simulink model "BiCopter_Landing"  (R2024a)
settings: Solver=ode4  StartTime=0.0  StopTime=20  FixedStep=0.005  RelTol=1e-3
values from neighbouring files (symbols this model uses):
  k = lqr(A,B,Q,R)    [K_Mat.m]    (also in R_good.mat = [-3.51546428725e-11 5.71513441117e-12 1000 1.44018719859e-11)
libraries: simulink_extras x6, shared6dof x3, fuzblock x3
settings Model: Creator=moham  LastModifiedBy=sepehrmahfar
settings OptimizationCC: ReuseModelBlockBuffer=off
settings RTWCC: GPUComputeCapability=3.5

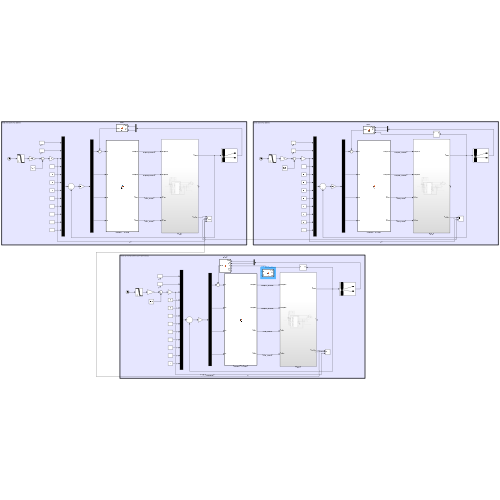
[thumbnail: Simulink's stored preview of the top-level diagram]
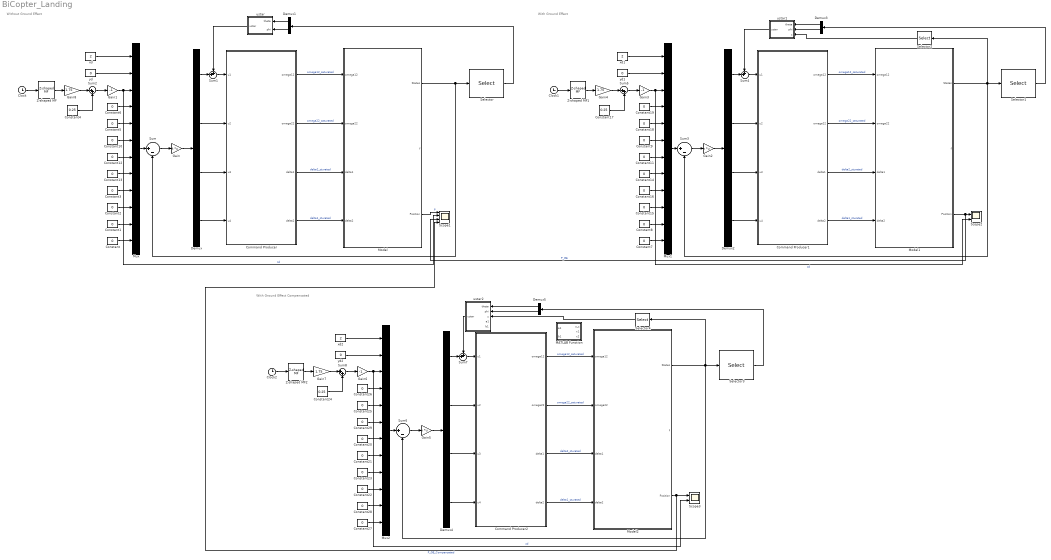
== system BiCopter_Landing ==
  note: Without Ground Effect
  note: With Ground Effect
  note: With Ground Effect Compensated
  Clock : Clock
  Clock1 : Clock
  Clock2 : Clock
  Command Producer : MATLAB Function  TreatAsAtomicUnit=on
  Command Producer1 : MATLAB Function  TreatAsAtomicUnit=on
  Command Producer2 : MATLAB Function  TreatAsAtomicUnit=on
  Constant{,1..3,5..16,18..23,25..29} (27 alike) : Constant  Value=0
  Constant17 : Constant  Value=0.25
  Constant24 : Constant  Value=0.25
  Constant4 : Constant  Value=0.25
  Demux : Demux
  Demux1 : Demux  Outputs=2
  Demux2 : Demux
  Demux3 : Demux  Outputs=2
  Demux4 : Demux
  Demux5 : Demux  Outputs=2
  Gain : Gain  Gain=k  Multiplication=Matrix(K*u)
  Gain1 : Gain  Gain=-1
  Gain2 : Gain  Gain=k  Multiplication=Matrix(K*u)
  Gain3 : Gain  Gain=-1
  Gain4 : Gain  Gain=1.75
  Gain5 : Gain  Gain=k  Multiplication=Matrix(K*u)
  Gain6 : Gain  Gain=-1
  Gain7 : Gain  Gain=1.75
  Gain8 : Gain  Gain=1.75
  MATLAB Function : MATLAB Function  TreatAsAtomicUnit=on
  Model : Subsystem
  Model1 : Subsystem
  Model2 : Subsystem
  Mux : Mux  Inputs=12
  Mux1 : Mux  Inputs=12
  Mux2 : Mux  Inputs=12
  Scope1 : Scope  NumInputPorts=4
  Scope2 : Scope  NumInputPorts=2
  Scope3 : Scope  NumInputPorts=2
  Selector : Selector  InputPortWidth=12  IndexOptions=Index vector (dialog)  Indices=[7 8]  OutputSizes=1
  Selector1 : Selector  InputPortWidth=12  IndexOptions=Index vector (dialog)  Indices=[7 8]  OutputSizes=1
  Selector2 : Selector  InputPortWidth=12  IndexOptions=Index vector (dialog)  Indices=3  OutputSizes=1
  Selector3 : Selector  InputPortWidth=12  IndexOptions=Index vector (dialog)  Indices=[7 8]  OutputSizes=1
  Selector4 : Selector  InputPortWidth=12  IndexOptions=Index vector (dialog)  Indices=3  OutputSizes=1
  Sum : Sum  Inputs=|+-
  Sum1 : Sum  Inputs=++|
  Sum2 : Sum  Inputs=|++
  Sum3 : Sum  Inputs=|+-
  Sum4 : Sum  Inputs=++|
  Sum5 : Sum  Inputs=|++
  Sum6 : Sum  Inputs=|+-
  Sum7 : Sum  Inputs=++|
  Sum8 : Sum  Inputs=|++
  Z-shaped MF : fuzblock/Membership  Functions/Z-shaped MF  a=10  b=15
  Z-shaped MF1 : fuzblock/Membership  Functions/Z-shaped MF  a=10  b=15
  Z-shaped MF2 : fuzblock/Membership  Functions/Z-shaped MF  a=10  b=15
  ustar : MATLAB Function  TreatAsAtomicUnit=on
  ustar1 : MATLAB Function  TreatAsAtomicUnit=on
  ustar2 : MATLAB Function  TreatAsAtomicUnit=on
  xd : Constant  Value=2
  xd1 : Constant  Value=2
  xd2 : Constant  Value=2
  yd : Constant  Value=0
  yd1 : Constant  Value=0
  yd2 : Constant  Value=0
  wires:
  Constant/1 -> Mux/12
  Model/1(States) -> Selector/1, Sum/2
  Mux/1 -> Sum/1
  Constant1/1 -> Mux/11
  Constant2/1 -> Mux/10
  Constant6/1 -> Mux/4
  Constant5/1 -> Mux/5
  Constant10/1 -> Mux/6
  Gain1/1 -> Scope1/2, Mux/3  "zd"
  Command Producer/4(delta2) -> Model/4(delta2)  "delta1_sturated"
  Command Producer/3(delta1) -> Model/3(delta1)  "delta2_sturated"
  Command Producer/2(omega22) -> Model/2(omega22)  "omega22_saturated"
  Command Producer/1(omega12) -> Model/1(omega12)  "omega12_saturated"
  Demux/4 -> Command Producer/4(u4)
  Demux/3 -> Command Producer/3(u3)
  Demux/2 -> Command Producer/2(u2)
  ustar/1(ustar) -> Sum1/1
  Constant12/1 -> Mux/7
  Constant13/1 -> Mux/8
  Sum/1 -> Gain/1
  Gain/1 -> Demux/1
  xd/1 -> Mux/1
  yd/1 -> Mux/2
  Selector/1 -> Demux1/1
  Demux1/2 -> ustar/2(phi)
  Demux1/1 -> ustar/1(theta)
  Model/3(Position) -> Scope1/1  "P"
  Constant3/1 -> Mux/9
  Sum1/1 -> Command Producer/1(u1)
  Demux/1 -> Sum1/2
  Gain8/1 -> Sum2/1
  Clock/1 -> Z-shaped MF/1
  Constant4/1 -> Sum2/2
  Z-shaped MF/1 -> Gain8/1
  Sum2/1 -> Gain1/1
  Demux3/1 -> ustar1/1(theta)
  Constant16/1 -> Mux1/9
  Gain2/1 -> Demux2/1
  Selector1/1 -> Demux3/1
  Model1/3(Position) -> Scope1/3, Scope2/1  "P_GE"
  xd1/1 -> Mux1/1
  Demux3/2 -> ustar1/2(phi)
  Constant19/1 -> Mux1/4
  Constant11/1 -> Mux1/7
  Command Producer1/4(delta2) -> Model1/4(delta2)  "delta1_sturated"
  ustar1/1(ustar) -> Sum4/1
  Constant18/1 -> Mux1/5
  Demux2/3 -> Command Producer1/3(u3)
  Constant7/1 -> Mux1/12
  Command Producer1/3(delta1) -> Model1/3(delta1)  "delta2_sturated"
  Gain3/1 -> Scope2/2, Mux1/3  "zd"
  Sum3/1 -> Gain2/1
  Command Producer1/2(omega22) -> Model1/2(omega22)  "omega22_saturated"
  Model1/1(States) -> Selector2/1, Selector1/1, Sum3/2
  Constant9/1 -> Mux1/6
  Constant8/1 -> Mux1/11
  yd1/1 -> Mux1/2
  Demux2/2 -> Command Producer1/2(u2)
  Constant15/1 -> Mux1/10
  Demux2/4 -> Command Producer1/4(u4)
  Mux1/1 -> Sum3/1
  Command Producer1/1(omega12) -> Model1/1(omega12)  "omega12_saturated"
  Demux2/1 -> Sum4/2
  Z-shaped MF1/1 -> Gain4/1
  Sum5/1 -> Gain3/1
  Gain4/1 -> Sum5/1
  Sum4/1 -> Command Producer1/1(u1)
  Constant17/1 -> Sum5/2
  Constant14/1 -> Mux1/8
  Clock1/1 -> Z-shaped MF1/1
  Selector2/1 -> ustar1/3(z)
  Z-shaped MF2/1 -> Gain7/1
  Constant26/1 -> Mux2/4
  Demux5/2 -> ustar2/2(phi)
  Constant27/1 -> Mux2/12
  Demux4/3 -> Command Producer2/3(u3)
  Sum6/1 -> Gain5/1
  Constant23/1 -> Mux2/9
  Gain6/1 -> Scope3/2, Mux2/3  "zd"
  Sum7/1 -> Command Producer2/1(u1)
  Gain5/1 -> Demux4/1
  Mux2/1 -> Sum6/1
  Constant25/1 -> Mux2/5
  yd2/1 -> Mux2/2
  Command Producer2/2(omega22) -> Model2/2(omega22)  "omega22_saturated"
  Clock2/1 -> Z-shaped MF2/1
  Demux4/4 -> Command Producer2/4(u4)
  Model2/1(States) -> Selector4/1, Selector3/1, Sum6/2
  Demux5/1 -> ustar2/1(theta)
  Constant28/1 -> Mux2/11
  Demux4/1 -> Sum7/2
  Gain7/1 -> Sum8/1
  Constant29/1 -> Mux2/6
  Constant24/1 -> Sum8/2
  Constant22/1 -> Mux2/10
  Command Producer2/1(omega12) -> Model2/1(omega12)  "omega12_saturated"
  Demux4/2 -> Command Producer2/2(u2)
  Sum8/1 -> Gain6/1
  Constant21/1 -> Mux2/8
  Constant20/1 -> Mux2/7
  Selector4/1 -> ustar2/3(z)
  ustar2/1(ustar) -> Sum7/1
  Selector3/1 -> Demux5/1
  Command Producer2/4(delta2) -> Model2/4(delta2)  "delta1_sturated"
  xd2/1 -> Mux2/1
  Command Producer2/3(delta1) -> Model2/3(delta1)  "delta2_sturated"
  Model2/3(Position) -> Scope3/1, Scope1/4  "P_GE_Compensated"

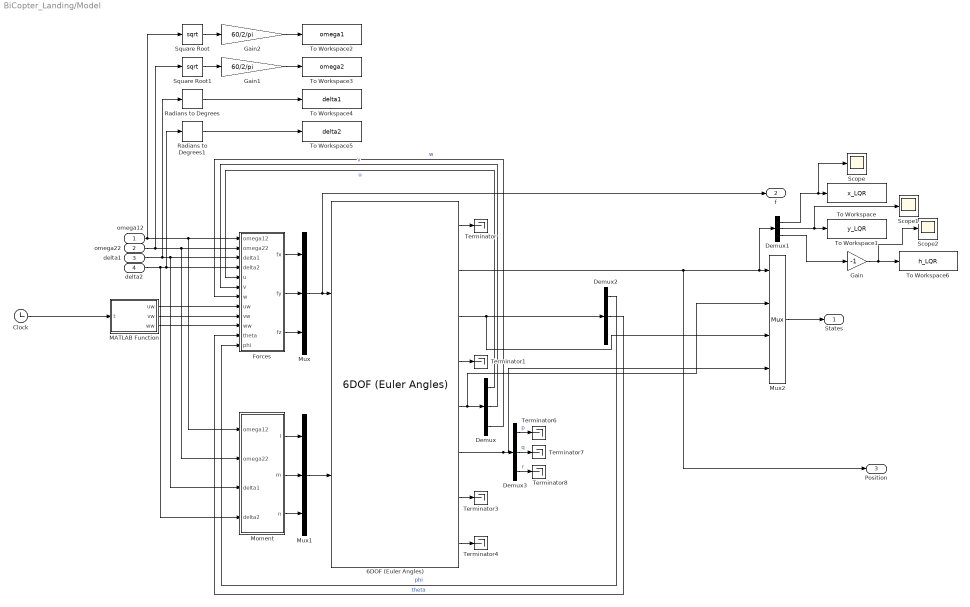
== system BiCopter_Landing/Model ==
  omega12 : Inport
  omega22 : Inport  Port=2
  delta1 : Inport  Port=3
  delta2 : Inport  Port=4
  6DOF (Euler Angles) : shared6dof/6DOF (Euler Angles)  units=Metric (MKS)  mtype=Fixed  rep=Euler Angles  xme_0=[2 0 -2]  Vm_0=[0 0 0]  eul_0=[0 0 0]  pm_0=[0 0 0]  mass_0=0.296  mass_e=0.5  mass_f=2.0  inertia=[0.0049, 0, -0.003675; 0, 0.0049, 0; -0.003675, 0, 0.0088]  inertia_e=eye(3)  inertia_f=2*eye(3)  k_quat=1.0  vre_flag=on  abi_flag=off  aMode=0  xme_statename=''  Vm_statename=''  eul_statename=''  quat_statename=''  pm_statename=''  mass_statename=''
  Clock : Clock
  Demux{,1..3} (4 alike) : Demux  Outputs=3
  Forces : MATLAB Function  TreatAsAtomicUnit=on
  Gain : Gain  Gain=-1
  Gain1 : Gain  Gain=60/2/pi
  Gain2 : Gain  Gain=60/2/pi
  MATLAB Function : MATLAB Function  TreatAsAtomicUnit=on
  Moment : MATLAB Function  TreatAsAtomicUnit=on
  Mux : Mux  Inputs=3
  Mux1 : Mux  Inputs=3
  Mux2 : Mux
  Radians to Degrees : simulink_extras/Transformations/Radians to Degrees
  Radians to Degrees1 : simulink_extras/Transformations/Radians to Degrees
  Scope : Scope
  Scope1 : Scope
  Scope2 : Scope
  Square Root : Sqrt
  Square Root1 : Sqrt
  Terminator{,1,3..4,6..8} (7 alike) : Terminator
  To Workspace : ToWorkspace  VariableName=x_LQR  SampleTime=-1
      settings: Save2DSignal=2-D array (concatenate along first dimension)
  To Workspace1 : ToWorkspace  VariableName=y_LQR  SampleTime=-1
      settings: Save2DSignal=2-D array (concatenate along first dimension)
  To Workspace2 : ToWorkspace  VariableName=omega1  SampleTime=-1
      settings: Save2DSignal=2-D array (concatenate along first dimension)
  To Workspace3 : ToWorkspace  VariableName=omega2  SampleTime=-1
      settings: Save2DSignal=2-D array (concatenate along first dimension)
  To Workspace4 : ToWorkspace  VariableName=delta1  SampleTime=-1
      settings: Save2DSignal=2-D array (concatenate along first dimension)
  To Workspace5 : ToWorkspace  VariableName=delta2  SampleTime=-1
      settings: Save2DSignal=2-D array (concatenate along first dimension)
  To Workspace6 : ToWorkspace  VariableName=h_LQR  SampleTime=-1
      settings: Save2DSignal=2-D array (concatenate along first dimension)
  States : Outport
  f : Outport  Port=2
  Position : Outport  Port=3
  wires:
  Moment/1(l) -> Mux1/1
  delta1/1 -> Moment/3(delta1), Forces/3(delta1), Radians to Degrees/1
  6DOF (Euler Angles)/5 -> Mux2/2, Demux/1
  Demux2/2 -> Forces/11(theta)  "theta"
  Mux/1 -> f/1, 6DOF (Euler Angles)/1
  6DOF (Euler Angles)/2 -> Position/1, Demux1/1, Mux2/1
  Forces/1(fx) -> Mux/1
  Forces/2(fy) -> Mux/2
  Mux1/1 -> 6DOF (Euler Angles)/2
  6DOF (Euler Angles)/4 -> Terminator1/1
  Demux/1 -> Forces/5(u)  "u"
  Clock/1 -> MATLAB Function/1(t)
  Demux2/1 -> Forces/12(phi)  "phi"
  Demux/2 -> Forces/6(v)  "v"
  omega12/1 -> Moment/1(omega12), Forces/1(omega12), Square Root/1
  6DOF (Euler Angles)/8 -> Terminator4/1
  6DOF (Euler Angles)/1 -> Terminator/1
  Moment/3(n) -> Mux1/3
  6DOF (Euler Angles)/7 -> Terminator3/1
  Moment/2(m) -> Mux1/2
  Forces/3(fz) -> Mux/3
  Demux/3 -> Forces/7(w)  "w"
  6DOF (Euler Angles)/3 -> Mux2/3, Demux2/1
  6DOF (Euler Angles)/6 -> Mux2/4, Demux3/1
  omega22/1 -> Moment/2(omega22), Forces/2(omega22), Square Root1/1
  delta2/1 -> Radians to Degrees1/1, Forces/4(delta2), Moment/4(delta2)
  Demux3/1 -> Terminator6/1  "p"
  Demux3/2 -> Terminator7/1  "q"
  Demux3/3 -> Terminator8/1  "r"
  Mux2/1 -> States/1
  Demux1/2 -> Scope1/1, To Workspace1/1
  Demux1/1 -> Scope/1, To Workspace/1
  Square Root/1 -> Gain2/1
  Square Root1/1 -> Gain1/1
  Radians to Degrees/1 -> To Workspace4/1
  Radians to Degrees1/1 -> To Workspace5/1
  Demux1/3 -> Gain/1
  Gain/1 -> Scope2/1, To Workspace6/1
  Gain1/1 -> To Workspace3/1
  Gain2/1 -> To Workspace2/1
  MATLAB Function/3(ww) -> Forces/10(ww)
  MATLAB Function/2(vw) -> Forces/9(vw)
  MATLAB Function/1(uw) -> Forces/8(uw)

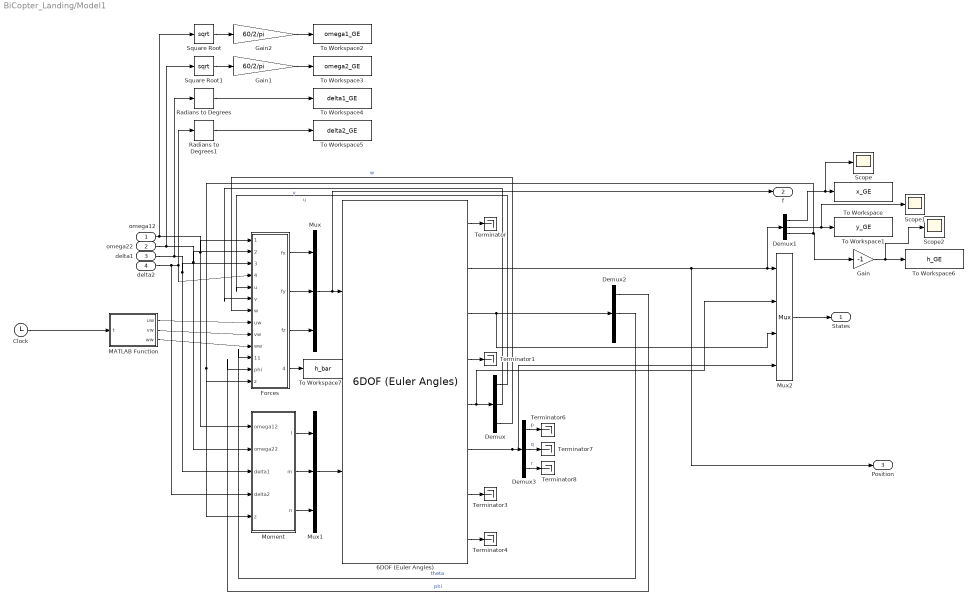
== system BiCopter_Landing/Model1 ==
  omega12 : Inport
  omega22 : Inport  Port=2
  delta1 : Inport  Port=3
  delta2 : Inport  Port=4
  6DOF (Euler Angles) : shared6dof/6DOF (Euler Angles)  units=Metric (MKS)  mtype=Fixed  rep=Euler Angles  xme_0=[2 0 -2]  Vm_0=[0 0 0]  eul_0=[0 0 0]  pm_0=[0 0 0]  mass_0=0.296  mass_e=0.5  mass_f=2.0  inertia=[0.0049, 0, -0.003675; 0, 0.0049, 0; -0.003675, 0, 0.0088]  inertia_e=eye(3)  inertia_f=2*eye(3)  k_quat=1.0  vre_flag=on  abi_flag=off  aMode=0  xme_statename=''  Vm_statename=''  eul_statename=''  quat_statename=''  pm_statename=''  mass_statename=''
  Clock : Clock
  Demux{,1..3} (4 alike) : Demux  Outputs=3
  Forces : MATLAB Function  TreatAsAtomicUnit=on
  Gain : Gain  Gain=-1
  Gain1 : Gain  Gain=60/2/pi
  Gain2 : Gain  Gain=60/2/pi
  MATLAB Function : MATLAB Function  TreatAsAtomicUnit=on
  Moment : MATLAB Function  TreatAsAtomicUnit=on
  Mux : Mux  Inputs=3
  Mux1 : Mux  Inputs=3
  Mux2 : Mux
  Radians to Degrees : simulink_extras/Transformations/Radians to Degrees
  Radians to Degrees1 : simulink_extras/Transformations/Radians to Degrees
  Scope : Scope
  Scope1 : Scope
  Scope2 : Scope
  Square Root : Sqrt
  Square Root1 : Sqrt
  Terminator{,1,3..4,6..8} (7 alike) : Terminator
  To Workspace : ToWorkspace  VariableName=x_GE  SampleTime=-1
      settings: Save2DSignal=2-D array (concatenate along first dimension)
  To Workspace1 : ToWorkspace  VariableName=y_GE  SampleTime=-1
      settings: Save2DSignal=2-D array (concatenate along first dimension)
  To Workspace2 : ToWorkspace  VariableName=omega1_GE  SampleTime=-1
      settings: Save2DSignal=2-D array (concatenate along first dimension)
  To Workspace3 : ToWorkspace  VariableName=omega2_GE  SampleTime=-1
      settings: Save2DSignal=2-D array (concatenate along first dimension)
  To Workspace4 : ToWorkspace  VariableName=delta1_GE  SampleTime=-1
      settings: Save2DSignal=2-D array (concatenate along first dimension)
  To Workspace5 : ToWorkspace  VariableName=delta2_GE  SampleTime=-1
      settings: Save2DSignal=2-D array (concatenate along first dimension)
  To Workspace6 : ToWorkspace  VariableName=h_GE  SampleTime=-1
      settings: Save2DSignal=2-D array (concatenate along first dimension)
  To Workspace7 : ToWorkspace  VariableName=h_bar  SaveFormat=Timeseries  SampleTime=-1
  States : Outport
  f : Outport  Port=2
  Position : Outport  Port=3
  wires:
  Moment/1(l) -> Mux1/1
  delta1/1 -> Moment/3(delta1), Forces/3(delta1), Radians to Degrees/1
  6DOF (Euler Angles)/5 -> Mux2/2, Demux/1
  Demux2/2 -> Forces/11(theta)  "theta"
  Mux/1 -> f/1, 6DOF (Euler Angles)/1
  6DOF (Euler Angles)/2 -> Position/1, Demux1/1, Mux2/1
  Forces/1(fx) -> Mux/1
  Forces/2(fy) -> Mux/2
  Mux1/1 -> 6DOF (Euler Angles)/2
  6DOF (Euler Angles)/4 -> Terminator1/1
  Demux/1 -> Forces/5(u)  "u"
  Clock/1 -> MATLAB Function/1(t)
  Demux2/1 -> Forces/12(phi)  "phi"
  Demux/2 -> Forces/6(v)  "v"
  omega12/1 -> Moment/1(omega12), Forces/1(omega12), Square Root/1
  6DOF (Euler Angles)/8 -> Terminator4/1
  6DOF (Euler Angles)/1 -> Terminator/1
  Moment/3(n) -> Mux1/3
  6DOF (Euler Angles)/7 -> Terminator3/1
  Moment/2(m) -> Mux1/2
  Forces/3(fz) -> Mux/3
  Demux/3 -> Forces/7(w)  "w"
  6DOF (Euler Angles)/3 -> Mux2/3, Demux2/1
  6DOF (Euler Angles)/6 -> Mux2/4, Demux3/1
  omega22/1 -> Moment/2(omega22), Forces/2(omega22), Square Root1/1
  delta2/1 -> Radians to Degrees1/1, Forces/4(delta2), Moment/4(delta2)
  Demux3/1 -> Terminator6/1  "p"
  Demux3/2 -> Terminator7/1  "q"
  Demux3/3 -> Terminator8/1  "r"
  Mux2/1 -> States/1
  Demux1/2 -> Scope1/1, To Workspace1/1
  Demux1/1 -> Scope/1, To Workspace/1
  Square Root/1 -> Gain2/1
  Square Root1/1 -> Gain1/1
  Radians to Degrees/1 -> To Workspace4/1
  Radians to Degrees1/1 -> To Workspace5/1
  Demux1/3 -> Moment/5(z), Forces/13(z), Gain/1
  Gain/1 -> Scope2/1, To Workspace6/1
  Gain1/1 -> To Workspace3/1
  Gain2/1 -> To Workspace2/1
  MATLAB Function/3(ww) -> Forces/10(ww)
  MATLAB Function/2(vw) -> Forces/9(vw)
  MATLAB Function/1(uw) -> Forces/8(uw)
  Forces/4(h_bar) -> To Workspace7/1

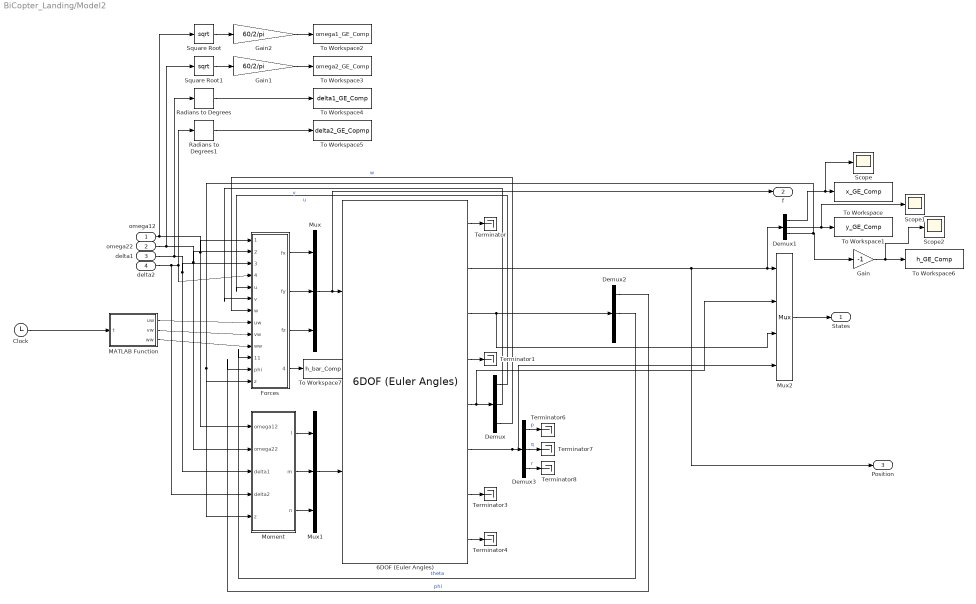
== system BiCopter_Landing/Model2 ==
  omega12 : Inport
  omega22 : Inport  Port=2
  delta1 : Inport  Port=3
  delta2 : Inport  Port=4
  6DOF (Euler Angles) : shared6dof/6DOF (Euler Angles)  units=Metric (MKS)  mtype=Fixed  rep=Euler Angles  xme_0=[2 0 -2]  Vm_0=[0 0 0]  eul_0=[0 0 0]  pm_0=[0 0 0]  mass_0=0.296  mass_e=0.5  mass_f=2.0  inertia=[0.0049, 0, -0.003675; 0, 0.0049, 0; -0.003675, 0, 0.0088]  inertia_e=eye(3)  inertia_f=2*eye(3)  k_quat=1.0  vre_flag=on  abi_flag=off  aMode=0  xme_statename=''  Vm_statename=''  eul_statename=''  quat_statename=''  pm_statename=''  mass_statename=''
  Clock : Clock
  Demux{,1..3} (4 alike) : Demux  Outputs=3
  Forces : MATLAB Function  TreatAsAtomicUnit=on
  Gain : Gain  Gain=-1
  Gain1 : Gain  Gain=60/2/pi
  Gain2 : Gain  Gain=60/2/pi
  MATLAB Function : MATLAB Function  TreatAsAtomicUnit=on
  Moment : MATLAB Function  TreatAsAtomicUnit=on
  Mux : Mux  Inputs=3
  Mux1 : Mux  Inputs=3
  Mux2 : Mux
  Radians to Degrees : simulink_extras/Transformations/Radians to Degrees
  Radians to Degrees1 : simulink_extras/Transformations/Radians to Degrees
  Scope : Scope
  Scope1 : Scope
  Scope2 : Scope
  Square Root : Sqrt
  Square Root1 : Sqrt
  Terminator{,1,3..4,6..8} (7 alike) : Terminator
  To Workspace : ToWorkspace  VariableName=x_GE_Comp  SampleTime=-1
      settings: Save2DSignal=2-D array (concatenate along first dimension)
  To Workspace1 : ToWorkspace  VariableName=y_GE_Comp  SampleTime=-1
      settings: Save2DSignal=2-D array (concatenate along first dimension)
  To Workspace2 : ToWorkspace  VariableName=omega1_GE_Comp  SampleTime=-1
      settings: Save2DSignal=2-D array (concatenate along first dimension)
  To Workspace3 : ToWorkspace  VariableName=omega2_GE_Comp  SampleTime=-1
      settings: Save2DSignal=2-D array (concatenate along first dimension)
  To Workspace4 : ToWorkspace  VariableName=delta1_GE_Comp  SampleTime=-1
      settings: Save2DSignal=2-D array (concatenate along first dimension)
  To Workspace5 : ToWorkspace  VariableName=delta2_GE_Copmp  SampleTime=-1
      settings: Save2DSignal=2-D array (concatenate along first dimension)
  To Workspace6 : ToWorkspace  VariableName=h_GE_Comp  SampleTime=-1
      settings: Save2DSignal=2-D array (concatenate along first dimension)
  To Workspace7 : ToWorkspace  VariableName=h_bar_Comp  SaveFormat=Timeseries  SampleTime=-1
  States : Outport
  f : Outport  Port=2
  Position : Outport  Port=3
  wires:
  Moment/1(l) -> Mux1/1
  delta1/1 -> Moment/3(delta1), Forces/3(delta1), Radians to Degrees/1
  6DOF (Euler Angles)/5 -> Mux2/2, Demux/1
  Demux2/2 -> Forces/11(theta)  "theta"
  Mux/1 -> f/1, 6DOF (Euler Angles)/1
  6DOF (Euler Angles)/2 -> Position/1, Demux1/1, Mux2/1
  Forces/1(fx) -> Mux/1
  Forces/2(fy) -> Mux/2
  Mux1/1 -> 6DOF (Euler Angles)/2
  6DOF (Euler Angles)/4 -> Terminator1/1
  Demux/1 -> Forces/5(u)  "u"
  Clock/1 -> MATLAB Function/1(t)
  Demux2/1 -> Forces/12(phi)  "phi"
  Demux/2 -> Forces/6(v)  "v"
  omega12/1 -> Moment/1(omega12), Forces/1(omega12), Square Root/1
  6DOF (Euler Angles)/8 -> Terminator4/1
  6DOF (Euler Angles)/1 -> Terminator/1
  Moment/3(n) -> Mux1/3
  6DOF (Euler Angles)/7 -> Terminator3/1
  Moment/2(m) -> Mux1/2
  Forces/3(fz) -> Mux/3
  Demux/3 -> Forces/7(w)  "w"
  6DOF (Euler Angles)/3 -> Mux2/3, Demux2/1
  6DOF (Euler Angles)/6 -> Mux2/4, Demux3/1
  omega22/1 -> Moment/2(omega22), Forces/2(omega22), Square Root1/1
  delta2/1 -> Radians to Degrees1/1, Forces/4(delta2), Moment/4(delta2)
  Demux3/1 -> Terminator6/1  "p"
  Demux3/2 -> Terminator7/1  "q"
  Demux3/3 -> Terminator8/1  "r"
  Mux2/1 -> States/1
  Demux1/2 -> Scope1/1, To Workspace1/1
  Demux1/1 -> Scope/1, To Workspace/1
  Square Root/1 -> Gain2/1
  Square Root1/1 -> Gain1/1
  Radians to Degrees/1 -> To Workspace4/1
  Radians to Degrees1/1 -> To Workspace5/1
  Demux1/3 -> Moment/5(z), Forces/13(z), Gain/1
  Gain/1 -> Scope2/1, To Workspace6/1
  Gain1/1 -> To Workspace3/1
  Gain2/1 -> To Workspace2/1
  MATLAB Function/3(ww) -> Forces/10(ww)
  MATLAB Function/2(vw) -> Forces/9(vw)
  MATLAB Function/1(uw) -> Forces/8(uw)
  Forces/4(h_bar) -> To Workspace7/1

== matlab function BiCopter_Landing/Model1/MATLAB Function ==
  data: t input; uw output; vw output; ww output
function [uw, vw, ww] = fcn(t)
uw = 0;
vw = 0;
ww = 0;

== matlab function BiCopter_Landing/Model1/Moment ==
  data: omega12 input; omega22 input; delta1 input; delta2 input; l output; m output; n output; z input
function [l, m, n] = fcn(omega12, omega22, delta1, delta2,z)
a = 0.225;
h_R = 0.0225;
R_Blade = 0.05;
h_bar = (-z+h_R)/(2.5*R_Blade);
b = 2.98e-6;
d = 1.14e-7;

if h_bar >= 2
    l = a*b*(omega12*cos(delta1)-omega22*cos(delta2)) + d*(-omega12*sin(delta1)+omega22*sin(delta2));
    m = -b*h_R*(omega12*sin(delta1)+omega22*sin(delta2));
    n = a*b*(omega12*sin(delta1)-omega22*sin(delta2)) + d*(omega12*cos(delta1)-omega22*cos(delta2));
else 
    l = (a*b*(omega12*cos(delta1)-omega22*cos(delta2)) + d*(-omega12*sin(delta1)+omega22*sin(delta2)))*(0.9926+0.03794*((2/h_bar)^2));
    m = (-b*h_R*(omega12*sin(delta1)+omega22*sin(delta2)))*(0.9926+0.03794*((2/h_bar)^2));
    n = (a*b*(omega12*sin(delta1)-omega22*sin(delta2)) + d*(omega12*cos(delta1)-omega22*cos(delta2)))*(0.9926+0.03794*((2/h_bar)^2));

end

== matlab function BiCopter_Landing/ustar1 ==
  data: theta input; phi input; ustar output; z input
function ustar  = fcn(theta, phi,z)
g = 9.81;
b = 2.98e-6;
m = 0.296;
h_R = 0.0225;
R_Blade = 0.1;
h_bar = (-z+h_R)/(2.5*R_Blade);
% ustar = m * g / b * cos(theta) * cos(phi)/(0.9926+0.03794*((2/h_bar)^2));
ustar = m * g / b * cos(theta) * cos(phi);

== matlab function BiCopter_Landing/Command Producer2 ==
  data: u1 input; omega12 output; omega22 output; delta1 output; delta2 output; u2 input; u3 input; u4 input
function [omega12, omega22, delta1, delta2] = fcn(u1, u2, u3, u4)
delta1 = atan2((u3+u4), (u1+u2));
delta2 = atan2((u3-u4), (u1-u2));
omega12 = 0.5 * (u1+u2) / cos(delta1);
omega22 = 0.5 * (u1-u2) / cos(delta2);
% a = 0.225;
% h = 0.0225;
% b = 2.98e-6;
% d = 1.14e-7;
% delta1 = atan2(b*h*(d*u2-b*a*u4) + ((d^2)+((b^2)*(a^2))*u3), b*h*(d*u4+b*a*u2) - h*(d^2)+((b^2)*(a^2))*u1);
% delta2 = atan2(b*h*(d*u2-b*a*u4) - ((d^2)+((b^2)*(a^2))*u3), b*h*(d*u4+b*a*u2) + h*(d^2)+((b^2)*(a^2))*u1);
% omega12 = ((b*h*(d*u2-b*a*u4) + ((d^2)+((b^2)*(a^2))*u3))^2) + (h^2)*((b*(d*u4 + b*a*u2) - ((d^2)+(b^2)*(a^2))*u1)^2) / (2*b*h*((d^2)+(b^2)*(a^2)));
% omega22 = ((b*h*(d*u2-b*a*u4) - ((d^2)+((b^2)*(a^2))*u3))^2) + (h^2)*((b*(d*u4 + b*a*u2) + ((d^2)+(b^2)*(a^2))*u1)^2) / (2*b*h*((d^2)+(b^2)*(a^2)));

== matlab function BiCopter_Landing/Model2/Forces ==
  data: omega12 input; omega22 input; delta1 input; delta2 input; u input; fx output; v input; w input; uw input; vw input; ww input; theta input; phi input; fy output; fz output; z input; h_bar output
function [fx, fy, fz, h_bar] = fcn(omega12, omega22, delta1, delta2, u, v, w, uw, vw, ww, theta, phi,z)
ua = u - uw;
va = v - vw;
wa = w - ww;
m = 0.296;
g = 9.81;
rho = 1.2682;
b = 2.98e-6;
s = 0.25;
CD = 0.32;
h_R = 0.0225;
R_Blade = 0.1;
h_bar = (-z+h_R)/(2.5*R_Blade);

if h_bar >= 2
    fx = -m*g*sin(theta) - 0.5*rho*s*CD*sqrt(ua^2+va^2+wa^2)*ua + b*(omega12*sin(delta1)+omega22*sin(delta2));
    fy = m*g*sin(phi)*cos(theta) - 0.5*rho*s*CD*sqrt(ua^2+va^2+wa^2)*va;
    fz = m*g*cos(phi)*cos(theta) - 0.5*rho*s*CD*sqrt(ua^2+va^2+wa^2)*wa - b*(omega12*cos(delta1)+omega22*cos(delta2));
else 
    fx = -m*g*sin(theta) - 0.5*rho*s*CD*sqrt(ua^2+va^2+wa^2)*ua + b*(omega12*sin(delta1)+omega22*sin(delta2))*(0.9926+0.03794*((2/h_bar)^2));
    fy = m*g*sin(phi)*cos(theta) - 0.5*rho*s*CD*sqrt(ua^2+va^2+wa^2)*va;
    fz = m*g*cos(phi)*cos(theta) - 0.5*rho*s*CD*sqrt(ua^2+va^2+wa^2)*wa - b*(omega12*cos(delta1)+omega22*cos(delta2))*(0.9926+0.03794*((2/h_bar)^2));
end

== matlab function BiCopter_Landing/Model2/MATLAB Function ==
  data: t input; uw output; vw output; ww output
function [uw, vw, ww] = fcn(t)
uw = 0;
vw = 0;
ww = 0;

== matlab function BiCopter_Landing/Model2/Moment ==
  data: omega12 input; omega22 input; delta1 input; delta2 input; l output; m output; n output; z input
function [l, m, n] = fcn(omega12, omega22, delta1, delta2,z)
a = 0.225;
h_R = 0.0225;
R_Blade = 0.05;
h_bar = (-z+h_R)/(2.5*R_Blade);
b = 2.98e-6;
d = 1.14e-7;

if h_bar >= 2
    l = a*b*(omega12*cos(delta1)-omega22*cos(delta2)) + d*(-omega12*sin(delta1)+omega22*sin(delta2));
    m = -b*h_R*(omega12*sin(delta1)+omega22*sin(delta2));
    n = a*b*(omega12*sin(delta1)-omega22*sin(delta2)) + d*(omega12*cos(delta1)-omega22*cos(delta2));
else 
    l = (a*b*(omega12*cos(delta1)-omega22*cos(delta2)) + d*(-omega12*sin(delta1)+omega22*sin(delta2)))*(0.9926+0.03794*((2/h_bar)^2));
    m = (-b*h_R*(omega12*sin(delta1)+omega22*sin(delta2)))*(0.9926+0.03794*((2/h_bar)^2));
    n = (a*b*(omega12*sin(delta1)-omega22*sin(delta2)) + d*(omega12*cos(delta1)-omega22*cos(delta2)))*(0.9926+0.03794*((2/h_bar)^2));

end

== matlab function BiCopter_Landing/ustar2 ==
  data: theta input; phi input; ustar output; z input; a1 input; b1 input
function ustar  = fcn(theta, phi,z, a1, b1)
g = 9.81;
b = 2.98e-6;
m = 0.296;
h_R = 0.0225;
R_Blade = 0.1;
h_bar = (-z+h_R)/(2.5*R_Blade);
ustar = m * g / b * cos(theta) * cos(phi)/((0.9926+a1)+(b1+0.03794)*((2/h_bar)^2));
% ustar = m * g / b * cos(theta) * cos(phi);

== matlab function BiCopter_Landing/MATLAB Function ==
  data: u_z input; a1 output; b1 output; x1 input; x2 input
function [a1,b1] = fcn(u_z,x1,x2)
x3 = 0;
x4 = 0;

A = [(0), (1.0), (0), (0); ((0.00032216216216216214529443779024687)*u_z*(x4 + (0.03794)))/((4.0)*x1 - (0.09))^3, -(0.34275675675675677200281942735249)*x2, -(0.000010067567567567567040451180945215)*u_z, -((0.000040270270270270268161804723780859)*u_z)/((4.0)*x1 - (0.09))^2; (0), (0), (0), (0); (0), (0), (0), (0)];
C = [1 0 0 0];

Ko = place(A',C',[-1 -2 -3 -4]);

== matlab function BiCopter_Landing/Model/Moment ==
  data: omega12 input; omega22 input; delta1 input; delta2 input; l output; m output; n output
function [l, m, n] = fcn(omega12, omega22, delta1, delta2)
a = 0.225;
h = 0.0225;
b = 2.98e-6;
d = 1.14e-7;
l = a*b*(omega12*cos(delta1)-omega22*cos(delta2)) + d*(-omega12*sin(delta1)+omega22*sin(delta2));
m = -b*h*(omega12*sin(delta1)+omega22*sin(delta2));
n = a*b*(omega12*sin(delta1)-omega22*sin(delta2)) + d*(omega12*cos(delta1)-omega22*cos(delta2));

== matlab function BiCopter_Landing/Model/Forces ==
  data: omega12 input; omega22 input; delta1 input; delta2 input; u input; fx output; v input; w input; uw input; vw input; ww input; theta input; phi input; fy output; fz output
function [fx, fy, fz] = fcn(omega12, omega22, delta1, delta2, u, v, w, uw, vw, ww, theta, phi)
ua = u - uw;
va = v - vw;
wa = w - ww;
m = 0.296;
g = 9.81;
rho = 1.2682;
s = 0.25;
CD = 0.32;
b = 2.98e-6;
fx = -m*g*sin(theta) - 0.5*rho*s*CD*sqrt(ua^2+va^2+wa^2)*ua + b*(omega12*sin(delta1)+omega22*sin(delta2));
fy = m*g*sin(phi)*cos(theta) - 0.5*rho*s*CD*sqrt(ua^2+va^2+wa^2)*va;
fz = m*g*cos(phi)*cos(theta) - 0.5*rho*s*CD*sqrt(ua^2+va^2+wa^2)*wa - b*(omega12*cos(delta1)+omega22*cos(delta2));

== matlab function BiCopter_Landing/Command Producer ==
  data: u1 input; omega12 output; omega22 output; delta1 output; delta2 output; u2 input; u3 input; u4 input
function [omega12, omega22, delta1, delta2] = fcn(u1, u2, u3, u4)
delta1 = atan2((u3+u4), (u1+u2));
delta2 = atan2((u3-u4), (u1-u2));
omega12 = 0.5 * (u1+u2) / cos(delta1);
omega22 = 0.5 * (u1-u2) / cos(delta2);
% a = 0.225;
% h = 0.0225;
% b = 2.98e-6;
% d = 1.14e-7;
% delta1 = atan2(b*h*(d*u2-b*a*u4) + ((d^2)+((b^2)*(a^2))*u3), b*h*(d*u4+b*a*u2) - h*(d^2)+((b^2)*(a^2))*u1);
% delta2 = atan2(b*h*(d*u2-b*a*u4) - ((d^2)+((b^2)*(a^2))*u3), b*h*(d*u4+b*a*u2) + h*(d^2)+((b^2)*(a^2))*u1);
% omega12 = ((b*h*(d*u2-b*a*u4) + ((d^2)+((b^2)*(a^2))*u3))^2) + (h^2)*((b*(d*u4 + b*a*u2) - ((d^2)+(b^2)*(a^2))*u1)^2) / (2*b*h*((d^2)+(b^2)*(a^2)));
% omega22 = ((b*h*(d*u2-b*a*u4) - ((d^2)+((b^2)*(a^2))*u3))^2) + (h^2)*((b*(d*u4 + b*a*u2) + ((d^2)+(b^2)*(a^2))*u1)^2) / (2*b*h*((d^2)+(b^2)*(a^2)));

== matlab function BiCopter_Landing/Model/MATLAB Function ==
  data: t input; uw output; vw output; ww output
function [uw, vw, ww] = fcn(t)
uw = 0;
vw = 0;
ww = 0;

== matlab function BiCopter_Landing/ustar ==
  data: theta input; phi input; ustar output
function ustar  = fcn(theta, phi)
g = 9.81;
b = 2.98e-6;
m = 0.296;
ustar = m * g / b * cos(theta) * cos(phi);

== matlab function BiCopter_Landing/Command Producer1 ==
  data: u1 input; omega12 output; omega22 output; delta1 output; delta2 output; u2 input; u3 input; u4 input
function [omega12, omega22, delta1, delta2] = fcn(u1, u2, u3, u4)
delta1 = atan2((u3+u4), (u1+u2));
delta2 = atan2((u3-u4), (u1-u2));
omega12 = 0.5 * (u1+u2) / cos(delta1);
omega22 = 0.5 * (u1-u2) / cos(delta2);
% a = 0.225;
% h = 0.0225;
% b = 2.98e-6;
% d = 1.14e-7;
% delta1 = atan2(b*h*(d*u2-b*a*u4) + ((d^2)+((b^2)*(a^2))*u3), b*h*(d*u4+b*a*u2) - h*(d^2)+((b^2)*(a^2))*u1);
% delta2 = atan2(b*h*(d*u2-b*a*u4) - ((d^2)+((b^2)*(a^2))*u3), b*h*(d*u4+b*a*u2) + h*(d^2)+((b^2)*(a^2))*u1);
% omega12 = ((b*h*(d*u2-b*a*u4) + ((d^2)+((b^2)*(a^2))*u3))^2) + (h^2)*((b*(d*u4 + b*a*u2) - ((d^2)+(b^2)*(a^2))*u1)^2) / (2*b*h*((d^2)+(b^2)*(a^2)));
% omega22 = ((b*h*(d*u2-b*a*u4) - ((d^2)+((b^2)*(a^2))*u3))^2) + (h^2)*((b*(d*u4 + b*a*u2) + ((d^2)+(b^2)*(a^2))*u1)^2) / (2*b*h*((d^2)+(b^2)*(a^2)));

== matlab function BiCopter_Landing/Model1/Forces ==
  data: omega12 input; omega22 input; delta1 input; delta2 input; u input; fx output; v input; w input; uw input; vw input; ww input; theta input; phi input; fy output; fz output; z input; h_bar output
function [fx, fy, fz, h_bar] = fcn(omega12, omega22, delta1, delta2, u, v, w, uw, vw, ww, theta, phi,z)
ua = u - uw;
va = v - vw;
wa = w - ww;
m = 0.296;
g = 9.81;
rho = 1.2682;
b = 2.98e-6;
s = 0.25;
CD = 0.32;
h_R = 0.0225;
R_Blade = 0.1;
h_bar = (-z+h_R)/(2.5*R_Blade);

if h_bar >= 2
    fx = -m*g*sin(theta) - 0.5*rho*s*CD*sqrt(ua^2+va^2+wa^2)*ua + b*(omega12*sin(delta1)+omega22*sin(delta2));
    fy = m*g*sin(phi)*cos(theta) - 0.5*rho*s*CD*sqrt(ua^2+va^2+wa^2)*va;
    fz = m*g*cos(phi)*cos(theta) - 0.5*rho*s*CD*sqrt(ua^2+va^2+wa^2)*wa - b*(omega12*cos(delta1)+omega22*cos(delta2));
else 
    fx = -m*g*sin(theta) - 0.5*rho*s*CD*sqrt(ua^2+va^2+wa^2)*ua + b*(omega12*sin(delta1)+omega22*sin(delta2))*(0.9926+0.03794*((2/h_bar)^2));
    fy = m*g*sin(phi)*cos(theta) - 0.5*rho*s*CD*sqrt(ua^2+va^2+wa^2)*va;
    fz = m*g*cos(phi)*cos(theta) - 0.5*rho*s*CD*sqrt(ua^2+va^2+wa^2)*wa - b*(omega12*cos(delta1)+omega22*cos(delta2))*(0.9926+0.03794*((2/h_bar)^2));
end
